simulink model "ISC_laboratorio_02_03_02"  (R2019a)
settings: Solver=FixedStepAuto  StartTime=0.0  StopTime=10.0  RelTol=1e-3
undefined symbols (not defined in the file): x0
settings Model: Creator=guilh  LastModifiedBy=guilh
settings DataIOCC: SaveOutput=off  ReturnWorkspaceOutputs=off  TimeSaveName=t

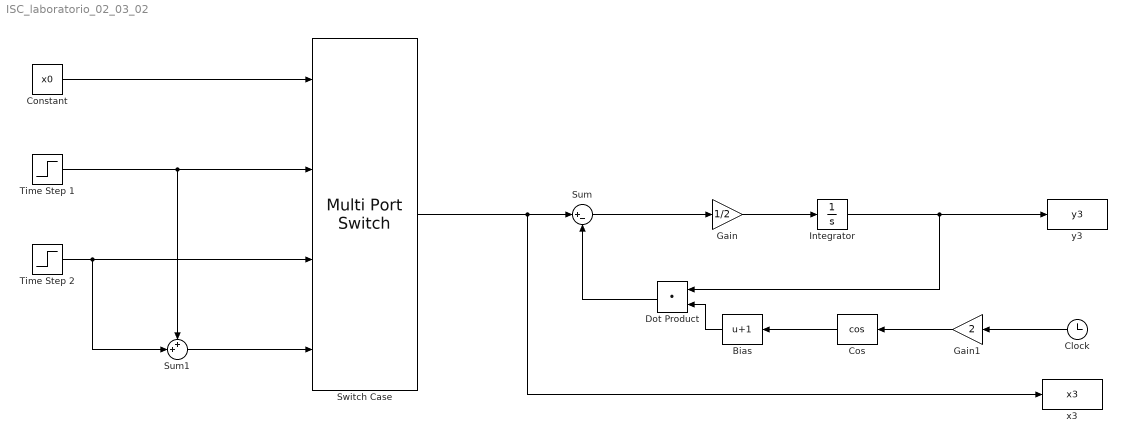
== system ISC_laboratorio_02_03_02 ==
  Bias : Bias  Bias=1
  Clock : Clock
  Constant : Constant  Value=x0
  Cos : Trigonometry  Operator=cos
  Dot Product : DotProduct  InputSameDT=on  OutDataTypeStr=Inherit: Inherit via internal rule
  Gain : Gain  Gain=1/2
  Gain1 : Gain  Gain=2
  Integrator : Integrator
  Sum : Sum  Inputs=|+-
  Sum1 : Sum  Inputs=++|
  Switch Case : MultiPortSwitch
  Time Step 1 : Step  SampleTime=0
  Time Step 2 : Step  Time=2  SampleTime=0
  x3 : ToWorkspace  VariableName=x3  SampleTime=-1
  y3 : ToWorkspace  VariableName=y3  SampleTime=-1
  wires:
  Integrator/1 -> Dot Product/1, y3/1
  Clock/1 -> Gain1/1
  Cos/1 -> Bias/1
  Bias/1 -> Dot Product/2
  Gain1/1 -> Cos/1
  Time Step 1/1 -> Sum1/1, Switch Case/2
  Constant/1 -> Switch Case/1
  Sum1/1 -> Switch Case/4
  Time Step 2/1 -> Sum1/2, Switch Case/3
  Gain/1 -> Integrator/1
  Sum/1 -> Gain/1
  Switch Case/1 -> x3/1, Sum/1
  Dot Product/1 -> Sum/2
